simulink model "test_track2"  (R2023a)
settings: Solver=VariableStepAuto  StartTime=0.0  StopTime=600  RelTol=1e-3
settings Model: Creator=lpb10197  LastModifiedBy=lpb10197
settings DebuggingCC: UnconnectedInputMsg=warning  UnconnectedOutputMsg=warning  UnconnectedLineMsg=warning
settings ModelReferenceCC: EnableRefExpFcnMdlSchedulingChecks=on
settings RTWCC: DLArmComputeVersion=19.05

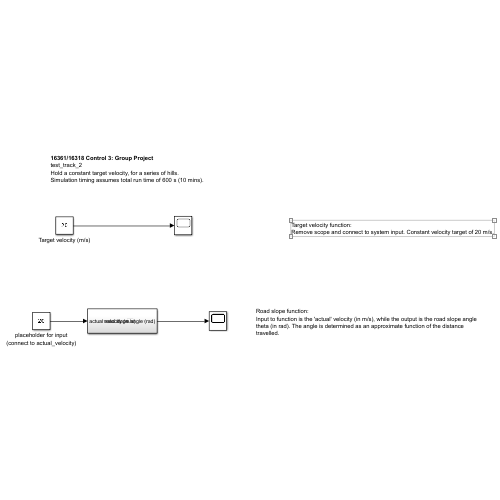
[thumbnail: Simulink's stored preview of the top-level diagram]
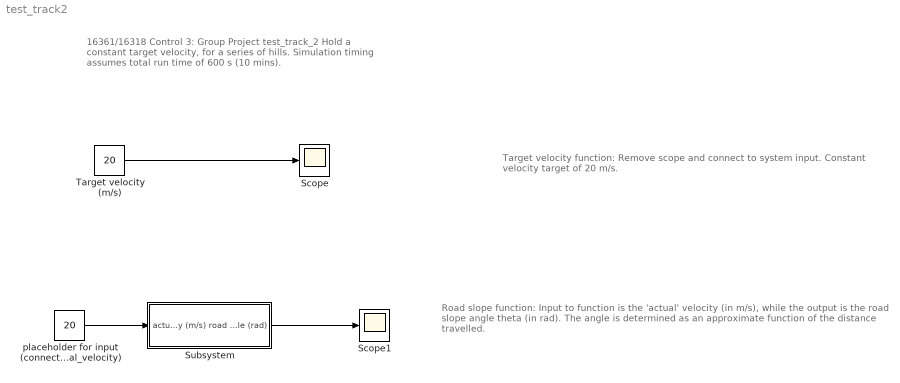
== system test_track2 ==
  note: Road slope function:
      | Input to function is the 'actual' velocity (in m/s), while the output is the road slope angle theta (in rad). The angle is determined as an approximate function of the distance travelled.
  note: Target velocity function:
      | Remove scope and connect to system input. Constant velocity target of 20 m/s.
  note: 16361/16318 Control 3: Group Project
      | test_track_2
      | Hold a constant target velocity, for a series of hills.
      | Simulation timing assumes total run time of 600 s (10 mins).
  Scope : Scope
  Scope1 : Scope
  Subsystem : Subsystem
  Target velocity (m/s) : Constant  Value=20
  placeholder for input (connect to actual_velocity) : Constant  Value=20
  wires:
  Subsystem/1(road slope angle (rad)) -> Scope1/1
  Target velocity (m/s)/1 -> Scope/1
  placeholder for input (connect to actual_velocity)/1 -> Subsystem/1(actual velocity (m/s))

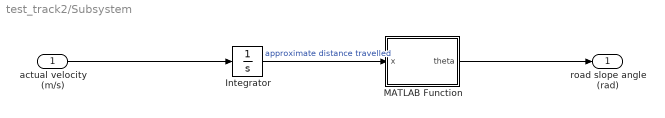
== system test_track2/Subsystem ==
  actual velocity (m/s) : Inport
  Integrator : Integrator
  MATLAB Function : MATLAB Function  TreatAsAtomicUnit=on
  road slope angle (rad) : Outport
  wires:
  MATLAB Function/1(theta) -> road slope angle (rad)/1
  actual velocity (m/s)/1 -> Integrator/1
  Integrator/1 -> MATLAB Function/1(x)  "approximate distance travelled"

== matlab function test_track2/Subsystem/MATLAB Function ==
  data: x input; theta output
function theta = fcn(x)

theta = pi/18*exp(0.0001*x)*sin(0.0015*x)*cos(0.001*x)+pi/18;
